simulink model "exp_07_b"  (R2018b)
settings: Solver=VariableStepAuto  StartTime=0.0  StopTime=10.0  RelTol=1e-3
settings Model: Creator=student  LastModifiedBy=student

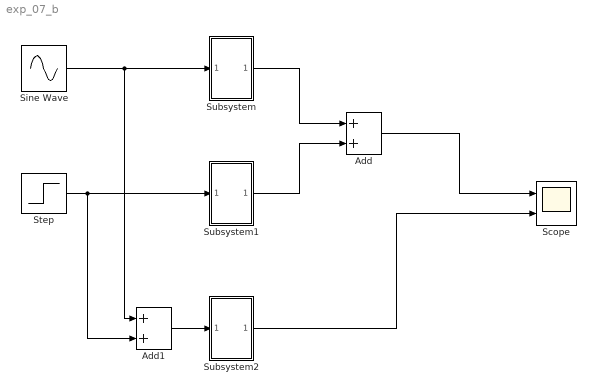
== system exp_07_b ==
  Add : Sum
  Add1 : Sum
  Scope : Scope  NumInputPorts=2
  Sine Wave : Sin  SampleTime=0
  Step : Step  SampleTime=0
  Subsystem : Subsystem
  Subsystem1 : Subsystem
  Subsystem2 : Subsystem
  wires:
  Sine Wave/1 -> Add1/1, Subsystem/1(In1)
  Step/1 -> Add1/2, Subsystem1/1(In1)
  Subsystem/1(Out1) -> Add/1
  Subsystem1/1(Out1) -> Add/2
  Add/1 -> Scope/1
  Add1/1 -> Subsystem2/1(In1)
  Subsystem2/1(Out1) -> Scope/2

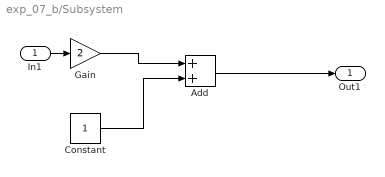
== system exp_07_b/Subsystem ==
  In1 : Inport
  Add : Sum
  Constant : Constant
  Gain : Gain  Gain=2
  Out1 : Outport
  wires:
  Gain/1 -> Add/1
  Add/1 -> Out1/1
  Constant/1 -> Add/2
  In1/1 -> Gain/1

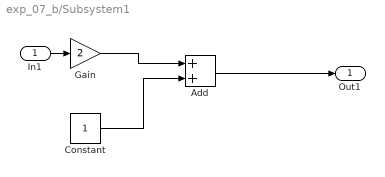
== system exp_07_b/Subsystem1 ==
  In1 : Inport
  Add : Sum
  Constant : Constant
  Gain : Gain  Gain=2
  Out1 : Outport
  wires:
  Gain/1 -> Add/1
  Add/1 -> Out1/1
  Constant/1 -> Add/2
  In1/1 -> Gain/1

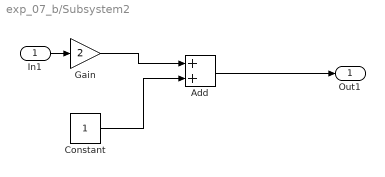
== system exp_07_b/Subsystem2 ==
  In1 : Inport
  Add : Sum
  Constant : Constant
  Gain : Gain  Gain=2
  Out1 : Outport
  wires:
  Gain/1 -> Add/1
  Add/1 -> Out1/1
  Constant/1 -> Add/2
  In1/1 -> Gain/1
